simulink subsystem "AnglesToPosition"  (R2019b)
settings: Solver=VariableStepAuto  StartTime=0.0  StopTime=10.0  RelTol=1e-3
settings Model: Creator=toons  LastModifiedBy=toons

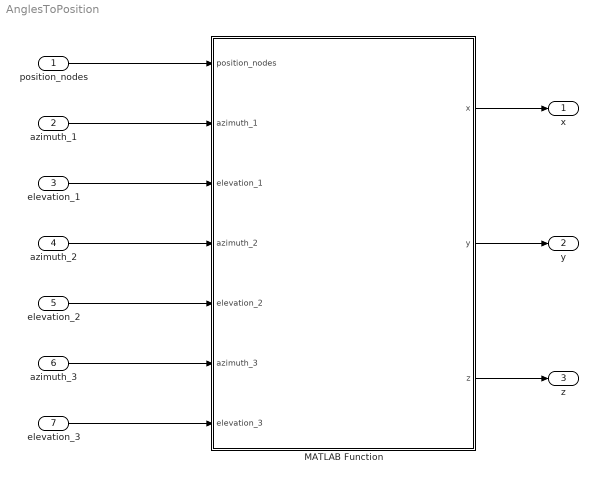
== system AnglesToPosition ==
  position_nodes : Inport
  azimuth_1 : Inport  Port=2
  elevation_1 : Inport  Port=3
  azimuth_2 : Inport  Port=4
  elevation_2 : Inport  Port=5
  azimuth_3 : Inport  Port=6
  elevation_3 : Inport  Port=7
  MATLAB Function : MATLAB Function  TreatAsAtomicUnit=on
  x : Outport
  y : Outport  Port=2
  z : Outport  Port=3
  wires:
  elevation_2/1 -> MATLAB Function/5(elevation_2)
  azimuth_2/1 -> MATLAB Function/4(azimuth_2)
  elevation_1/1 -> MATLAB Function/3(elevation_1)
  azimuth_1/1 -> MATLAB Function/2(azimuth_1)
  position_nodes/1 -> MATLAB Function/1(position_nodes)
  azimuth_3/1 -> MATLAB Function/6(azimuth_3)
  elevation_3/1 -> MATLAB Function/7(elevation_3)
  MATLAB Function/2(y) -> y/1
  MATLAB Function/1(x) -> x/1
  MATLAB Function/3(z) -> z/1

== matlab function AnglesToPosition/MATLAB Function ==
  data: position_nodes input; x output; azimuth_1 input; elevation_1 input; azimuth_2 input; elevation_2 input; azimuth_3 input; elevation_3 input; y output; z output
function [x,y,z] = AnglesToPosition(position_nodes, azimuth_1, ...
    elevation_1, azimuth_2, elevation_2, azimuth_3, elevation_3)

directions = [azimuth_1, elevation_1; azimuth_2, elevation_2; ...
    azimuth_3, elevation_3];
vectors = AnglesToVectors(position_nodes, directions);
[x,y,z] = VectorsToIntersection(vectors);

end
